simulink model "PMSMModel"  (R2022a)
settings: Solver=ode1  StartTime=0.0  StopTime=10.0  FixedStep=1e-5  RelTol=1e-3
values from neighbouring files (symbols this model uses):
  A = [0 -Lq  ; Ld 0 ]    [PMSMParameters.m]
  C0 = 3.53*10.^-1    (= 0.353)    [PMSMParameters.m]
  F = 1.57*10.^-3    (= 0.00157)    [PMSMParameters.m]
  J = 5.21*10.^-3    (= 0.00521)    [PMSMParameters.m]
  L = [Ld 0 ; 0 Lq ]    [PMSMParameters.m]
  P = 2    [PMSMParameters.m]
  phif = [0 ; pf]    [PMSMParameters.m]
  R = [Rs 0; 0 Rs ]    [PMSMParameters.m]
settings Model: Creator=ZinouAb  LastModifiedBy=ZinouAb
settings ModelReferenceCC: EnableRefExpFcnMdlSchedulingChecks=off
settings RTWCC: Description=Generic Real-Time Target

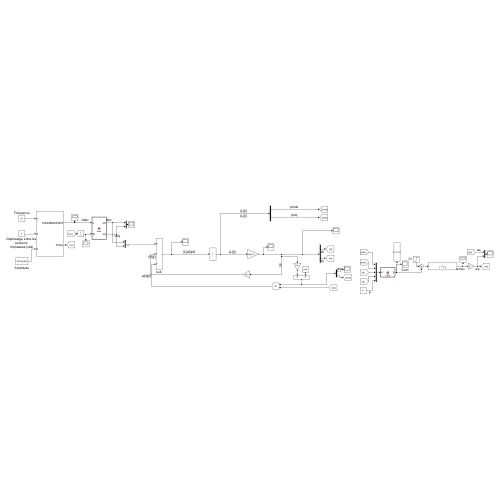
[thumbnail: Simulink's stored preview of the top-level diagram]
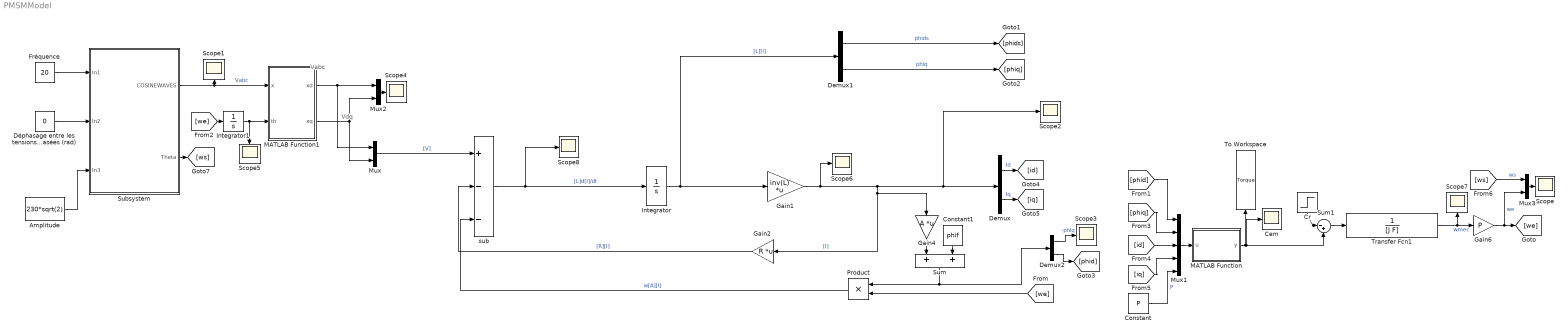
== system PMSMModel ==
  note: Vdq
  note: Vabc
  Amplitude : Constant  Value=230*sqrt(2)
  Cem : Scope
  Constant : Constant  Value=P
  Constant1 : Constant  Value=phif
  Cr : Step  Time=4  After=1+C0  SampleTime=0
  Demux : Demux  Outputs=2
  Demux1 : Demux  Outputs=2
  Demux2 : Demux  Outputs=2
  Déphasage entre les tensions triphasées (rad) : Constant  Value=0
  Fréquence : Constant  Value=20
  Gain1 : Gain  Gain=inv(L)  Multiplication=Matrix(K*u)
  Gain2 : Gain  Gain=R  Multiplication=Matrix(K*u)
  Gain4 : Gain  Gain=A  Multiplication=Matrix(K*u)
  Gain6 : Gain  Gain=P
  Integrator : Integrator
  Integrator1 : Integrator
  MATLAB Function : MATLAB Function  TreatAsAtomicUnit=on
  MATLAB Function1 : MATLAB Function  TreatAsAtomicUnit=on
  Mux : Mux  Inputs=2
  Mux1 : Mux  Inputs=5
  Mux2 : Mux  Inputs=2
  Mux3 : Mux  Inputs=2
  Product : Product
  Scope{,1..8} (9 alike) : Scope
  Subsystem : Subsystem
  Sum : Sum
  Sum1 : Sum  Inputs=|-+
  To Workspace : ToWorkspace  VariableName=Torque  SaveFormat=Timeseries  SampleTime=-1
  Transfer Fcn1 : TransferFcn  Denominator=[J F]
  sub : Sum  Inputs=+--
  wires:
  Integrator1/1 -> Scope5/1, MATLAB Function1/2(th)
  Subsystem/1(COSINEWAVES) -> MATLAB Function1/1(x), Scope1/1  "Vabc"
  Mux2/1 -> Scope4/1
  Fréquence/1 -> Subsystem/1(In1)
  Déphasage entre les tensions triphasées (rad)/1 -> Subsystem/2(In2)
  MATLAB Function1/1(xd) -> Mux/1, Mux2/1
  MATLAB Function1/2(xq) -> Mux/2, Mux2/2
  [we] -> Integrator1/1
  Subsystem/2(Theta) -> [ws]
  Amplitude/1 -> Subsystem/3(In3)
  Mux/1 -> sub/1  "[V]"
  [we] -> Product/2
  Integrator/1 -> Gain1/1, Demux1/1  "[L][I]"
  [phiq] -> Mux1/2
  Demux/2 -> [iq]  "Iq"
  sub/1 -> Scope8/1, Integrator/1  "[L]d[I]/dt"
  Mux1/1 -> MATLAB Function/1(u)
  Demux2/1 -> Scope3/1  "-phiq"
  [ws] -> Mux3/1  "ws"
  Cr/1 -> Sum1/1
  Mux3/1 -> Scope/1
  Sum1/1 -> Transfer Fcn1/1
  Constant/1 -> Mux1/5  "P"
  Transfer Fcn1/1 -> Gain6/1, Scope7/1  "wmec"
  Gain6/1 -> Mux3/2, [we]  "we"
  [id] -> Mux1/3
  Constant1/1 -> Sum/2
  [phid] -> Mux1/1
  Gain4/1 -> Sum/1
  Product/1 -> sub/3  "w[A][I]"
  Demux1/2 -> [phiq]  "phiq"
  Demux/1 -> [id]  "Id"
  Gain2/1 -> sub/2  "[R][I]"
  MATLAB Function/1(y) -> Sum1/2, Cem/1, To Workspace/1
  [iq] -> Mux1/4
  Demux2/2 -> [phid]
  Demux1/1 -> [phids]  "phids"
  Gain1/1 -> Gain2/1, Gain4/1, Scope2/1, Demux/1, Scope6/1  "[I]"
  Sum/1 -> Product/1, Demux2/1

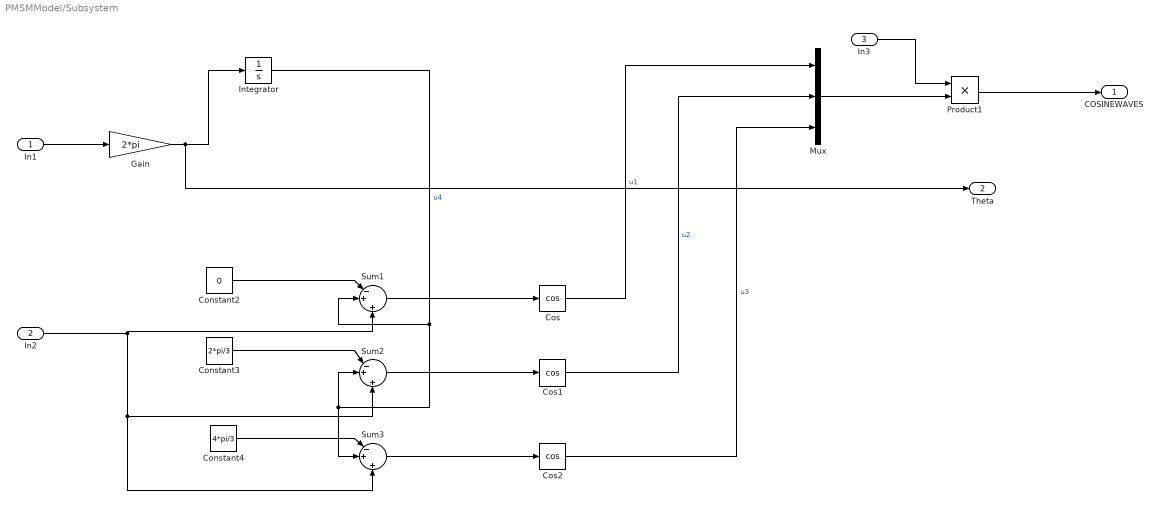
== system PMSMModel/Subsystem ==
  In1 : Inport
  In2 : Inport  Port=2
  In3 : Inport  Port=3
  Constant2 : Constant  Value=0
  Constant3 : Constant  Value=2*pi/3
  Constant4 : Constant  Value=4*pi/3
  Cos : Trigonometry  Operator=cos
  Cos1 : Trigonometry  Operator=cos
  Cos2 : Trigonometry  Operator=cos
  Gain : Gain  Gain=2*pi
  Integrator : Integrator
  Mux : Mux  Inputs=3
  Product1 : Product
  Sum1 : Sum  Inputs=|-+|+
  Sum2 : Sum  Inputs=|-+|+
  Sum3 : Sum  Inputs=|-+|+
  COSINEWAVES : Outport
  Theta : Outport  Port=2
  wires:
  Sum2/1 -> Cos1/1
  In2/1 -> Sum1/3, Sum3/3, Sum2/3
  Integrator/1 -> Sum3/2, Sum2/2, Sum1/2  "u4"
  Constant3/1 -> Sum2/1
  Sum3/1 -> Cos2/1
  Sum1/1 -> Cos/1
  Constant2/1 -> Sum1/1
  Constant4/1 -> Sum3/1
  Gain/1 -> Theta/1, Integrator/1
  In1/1 -> Gain/1
  Cos1/1 -> Mux/2  "u2"
  Cos/1 -> Mux/1  "u1"
  Cos2/1 -> Mux/3  "u3"
  In3/1 -> Product1/1
  Mux/1 -> Product1/2
  Product1/1 -> COSINEWAVES/1

== matlab function PMSMModel/MATLAB Function1 ==
  data: x input; xd output; xq output; th input
function [xd,xq] = Park(x,th)
% vd=(2/3)*(u1*cos(th)+u2*cos(th-2*pi/3)+u3*cos(th+2*pi/3));
% vq=(2/3)*(-u1*sin(th)-u2*sin(th-2*pi/3)-u3*sin(th+2*pi/3));
P=(2/3)*[ cos(th) cos(th-2*pi/3) cos(th+2*pi/3);
         -sin(th) -sin(th-2*pi/3) -sin(th+2*pi/3)  ];
prod=P*x;
xd=prod(1);
xq=prod(2);

== matlab function PMSMModel/MATLAB Function ==
  data: u input; y output
function y = CEM(u)

y =(3/2)*u(5)*(u(1)*u(4)-u(2)*u(3));
